simulink library "lib_Convection_SimpNatConvHeatXII"  (R2015a)
settings: Solver=ode45  StartTime=0.0  StopTime=10.0  RelTol=1e-3
settings Model: Creator=jlkratz  LastModifiedBy=jlkratz

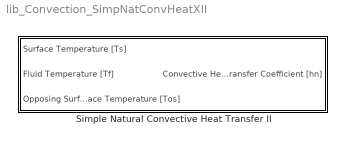
== system lib_Convection_SimpNatConvHeatXII ==
  Simple Natural Convective Heat Transfer II : Subsystem  mask(Simple Natural Convective Heat Transfer Block (T-SAT)){hcoeff_M=0.03, dTdes_M=1, BN_M=gcb}
      mask prompts: hcoeff_M "hcoeff_M - Convective heat transfer coefficient when W = Wdes and T = Tdes"; dTdes_M "dTdes_M - Design Ts - Tr (known data point)"; BN_M "BN_M - Block name"
      mask help:
      | This block models takes a simplistic apporach at modeling the natural convection heat transfer coefficient (hn). The equation for calculating the convective heat transfer coefficient is based on empirical models and attempts to correlate the heat transfer coefficient with the surface and fluid temperatures (Ts and Tr respectively).
      |
      | h = hcoeff * [0.5((Ts-Tf)+(Ts-Tos))/dTdes]^(0.25)
      |
      | In the equation above, (Ts-Tr)des is the temperautre difference of the surface and fluid when h = hcoeff. This block can accept various units but the units must be consistent.
      mask Help: web(which('Convection_TSAT_SimpNatConvHeatXII.html'),'-helpbrowser')

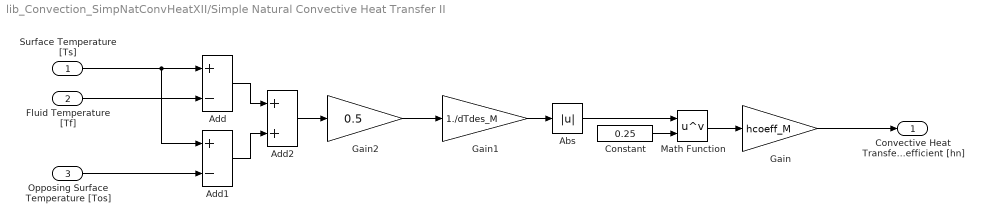
== system lib_Convection_SimpNatConvHeatXII/Simple Natural Convective Heat Transfer II ==
  "Surface Temperature [Ts] " : Inport
  Fluid Temperature [Tf] : Inport  Port=2
  Opposing Surface Temperature [Tos] : Inport  Port=3
  Abs : Abs
  Add : Sum  Inputs=+-
  Add1 : Sum  Inputs=+-
  Add2 : Sum
  Constant : Constant  Value=0.25
  Gain : Gain  Gain=hcoeff_M
  Gain1 : Gain  Gain=1./dTdes_M
  Gain2 : Gain  Gain=0.5
  Math Function : Math  Operator=pow  SaturateOnIntegerOverflow=on
  Convective Heat Transfer Coefficient [hn] : Outport
  wires:
  Gain2/1 -> Gain1/1
  Add2/1 -> Gain2/1
  Add1/1 -> Add2/2
  Add/1 -> Add2/1
  Opposing Surface Temperature [Tos]/1 -> Add1/2
  "Surface Temperature [Ts] "/1 -> Add/1, Add1/1
  Math Function/1 -> Gain/1
  Fluid Temperature [Tf]/1 -> Add/2
  Gain/1 -> Convective Heat Transfer Coefficient [hn]/1
  Constant/1 -> Math Function/2
  Abs/1 -> Math Function/1
  Gain1/1 -> Abs/1
